simulink model "RPBSIDblocks"  (Simulink 7.8)
settings: Solver=ode45  StartTime=0.0  StopTime=10.0  RelTol=1e-3
values from neighbouring files (symbols this model uses):
  Du = 164.831638116    [GUST2data.mat]
  Dy = [1.80356893973  0; 0  1.68127100115]    [GUST2data.mat]
undefined symbols (not defined in the file or in its folder): W
libraries: cstblocks x1
(part 2 of 2)

== matlab function RPBSID (VARX) FAST-ARRAY ==
  data: ON input double; RESET input double; Ws output double; Fs1 output double; Fs2 output double; U input double; Y input double size=2; Wn output double; Zn output double; W parameter double; Du parameter double; Dy parameter double; ERR output double
function [Ws,Fs1,Fs2,Wn,Zn,ERR] = rpbsid(ON,RESET,U,Y,W,Du,Dy)
%RPBSID Closed-loop recursive predictor-based subspace identification (VARX)

% Input definitions
% U input sample
% Y output sample
% W weight matrix (from workspace)
% Du input scaling matrix from sigscale (from workspace)
% Dy output scaling matric from sigscale (from workspace)

% Common paremeters
r = 1;         % number if inpuh
l = 2;         % number of outpuh
m = l+r;
n = 7;         % number of states
Ts = 0.05;      % sample time

% Parameters for identification
p = 50;        % past window
f = 50;        % future window
noD = 0;       % no direct feedtrough
weight = 0;    % apply transformation filter

% Parameters for adaptive filters
lambda1 = 0.999; % initial forgetting factor (~= 1 - 2/window)
lambda2 = 0.999; % initial forgetting factor (~= 1 - 2/window)
lambda3 = 0.999; % initial forgetting factor (~= 1 - 2/window)
ireg1 = 100;     % initial regularisation
ireg2 = 1e-6;    % initial regularisation
ireg3 = 1e-6;    % initial regularisation
reg1 = 1;        % initial regularisation
tol = 1e-4;      % tolerance setting for resque (fast array)

% Initialization
startA = 3;

% Initialize if needed
persistent Plk Glk Ylk VARX VARX1 LK Pcd Pabk ABK CD U1 Y1 X X1 Z eta w k start saw
if isempty(Plk) || RESET
    % Initialisation of Markov estimation problem
    if noD
        Plk = zeros((p+1)*m+1,2*m+1);
        Glk = zeros(p*m,m);
        Ylk = ones(1,m);
        VARX = zeros(l,p*m);
        VARX1 = zeros(l,p*m);
        Z = zeros((p+1)*m,1);
        eta = zeros((p+1)*m,m);
    else
        Plk = zeros((p+2)*m+1,2*m+1);
        Glk = zeros((p+1)*m,m);
        Ylk = ones(1,m);
        VARX = zeros(l,(p+1)*m);
        VARX1 = zeros(l,p*m);
        Z = zeros((p+2)*m,1);
        eta = zeros((p+2)*m,m);
    end
    saw = 0;
    
    % Initialisation of the LambdaKappa
    LK = zeros(f*l,m*p);
    
    % Initialisation the estimate of ABK
    Pabk = (1/sqrt(ireg2)).*eye(n+r+l);
    ABK = [zeros(n) zeros(n,r) zeros(n,l)];
    
    if noD
        % Initialisation the estimate of CD
        Pcd = (1/sqrt(ireg3)).*eye(n);
        CD = zeros(l,n);
    else
        % Initialisation the estimate of CD and e
        Pcd = (1/sqrt(ireg3)).*eye(n+r);
        CD = [zeros(l,n) zeros(l,r)];
    end

    % Store vectors for next iteration
    Y1 = zeros(l,1);
    U1 = zeros(r,1);
    X1 = zeros(n,1);
    X = zeros(n,1);
    
    % Frequency grid
    w = logspace(-1,1,300);
    k = 1;
    start = 1;
end

% Start RPBSID iff ON is set
if ON > 0.5
    
    % Scale input and output
    U = diag(1./diag(Du))*U;
    Y = diag(1./diag(Dy))*Y;
    
    if (start < 0.5) || (k >= p)
        % Solve Markov estimation problem recursively
        if noD
            [VARX,Z,Plk,eta,Glk,Ylk,saw,ERR] = fastQR(Z,[U1; Y1],Y,VARX,Plk,lambda1,tol,eta,ireg1,reg1,Glk,Ylk,saw);
            VARX1 = VARX;
        else
            [VARX,Z,Plk,eta,Glk,Ylk,saw,ERR] = fastQR(Z,[Y1; U],Y,VARX,Plk,lambda1,tol,eta,ireg1,reg1,Glk,Ylk,saw);
            VARX1 = VARX(:,l+1:p*m+l);
        end
    else
        ERR = 0;
    end
    
    if (start < 0.5) || (k >= startA*p)
        % Construction of LambdaKappa
        LK = zeros(f*l,p*m);
        if ~weight
            for i = 0:f-1
                for h = 0:p-i-1
                    LK(i*l+(1:l),(i+h)*m+(1:m)) = VARX1(:,h*m+(1:m));
                end
            end
        else
            for i = 0:f-1
                for h = 0:p-i-1
                    LK(i*l+(1:l),(i+h)*m+(1:m)) = VARX1(:,h*m+(1:m));
                end
                if i ~= 0
                    for j = 0:i-1
                        LK(i*l+(1:l),:) = LK(i*l+(1:l),:) + VARX1(:,(p-i+j)*m+r+(1:l))*LK(j*l+(1:l),:);
                    end
                end
            end
        end
        
        % The estimation of the state vector
        if noD
            X = W*LK*Z(m+1:(p+1)*m,1);
        else
            X = W*LK*Z(m+l+1:(p+1)*m+l,1);
        end
    end
    
    if (start < 0.5) || (k >= startA*p+1)
        % The estimation of the system matrices
        if noD
            [CD,Pcd] = inverseQR(X1,Y1,CD,Pcd,lambda2);
            R1 = Y1-CD*X1;
        else
            [CD,Pcd] = inverseQR([X1; U1],Y1,CD,Pcd,lambda2);
            R1 = Y1-CD*[X1; U1];
        end
        [ABK,Pabk] = inverseQR([X1; U1; R1],X,ABK,Pabk,lambda3);
    end
        
    % Store vectors and matrices for next iteration
    if (start < 0.5) || (k >= startA*p)
        X1 = X;
    end
    Y1 = Y;
    U1 = U;
else
    ERR = 0;
end

% Store state-space matrices
A = ABK(:,1:n);
B = ABK(:,n+1:n+r)*diag(1./diag(Du));
C = Dy*CD(:,1:n);
if noD
    D = zeros(l,r);
else
    D = Dy*CD(:,n+1:end)*diag(1./diag(Du));
end
K = ABK(:,n+r+1:n+r+l);

% Calculate damping and frequencies
[Wn,Zn] = damp(A,Ts);

% Calculate frequency response
Ws = w(k);
Fs = real(abs(C*((exp(sqrt(complex(-1))*Ts*Ws*2*pi).*eye(n) - A)\B)+D));
Ws = log10(Ws);
if Fs(1) < 1e-5
    Fs1 = -100;
else
    Fs1 = 20*log10(Fs(1));
end
if Fs(2) < 1e-5
    Fs2 = -100;
else
    Fs2 = 20*log10(Fs(2));
end

% Update counter
if k >= length(w)
    start = 0;
    k = 1;
else
    k = k+1;
end

end % END RPBSID


function [theta,z,M,eta,G,Y,saw,ERR] = fastQR(z,u,y,theta,M,lambda,tol,eta,ireg,reg,G,Y,saw)
%FASTQR Fast Recursive Least Squares (fast array QR)

n = length(u);
p = (length(z)/n - 1);
if M(1,1) == 0
    M(1,1) = 1;
    M(2:n+1,2:n+1) = diag((sqrt(lambda^p)/sqrt(ireg)).*ones(n,1));
    M(p*n+2:(p+1)*n+1,n+2:2*n+1) = diag((1/sqrt(ireg)).*ones(n,1));
end

% Do reg update
if saw > p-0.5;
    saw = 1;
    eta = [eta(n+1:end,:); sqrt((1-lambda^p)*reg).*eye(n)];
else
    saw = saw + 1;
    eta = [eta(n+1:end,:); zeros(n)];
end

G1 = M(2+n:end,1);
Y1 = M(1,1);
for j = 1:n
    M(1,1) = Y(1,j);
    M(2:end,2:end) = M(2:end,2:end);
    M(1,2:end) = eta(:,j)'*M(2:end,2:end);
    M(2:1+p*n,1) = G(1:end,j);
    M(2+p*n:end,1) = zeros(n,1);
    for i = 2:size(M,2)
        if i > (size(M,2)-n)
            % determine Givens rotation parameters
            if M(1,i) ~= 0
                % determine Givens rotation parameters
                rho = M(1,i)/M(1,1);
                c = sqrt(1+abs(rho)^2);
                
                % apply givens rotation using mixed-downdating
                M(:,1) = (M(:,1) + rho.*M(:,i))./c;
                M(:,i) = (-rho).*M(:,1) + c.*M(:,i);
            end
        else
            % determine hyperbolic rotation parameters
            if abs(M(i,i)) > abs(M(i,1))
                if M(i,1) ~= 0
                    % apply hyperbolic rotation using orthogonal-diagonal method
                    % method (numerically stable)
                    x1 = M(:,1) - M(:,i);
                    y1 = M(:,1) + M(:,i);
                    x2 = 0.5.*sqrt(-y1(i)/x1(i)).*x1;
                    y2 = 0.5.*sqrt(-x1(i)/y1(i)).*y1;
                    M(:,1) = x2 + y2;
                    M(:,i) = y2 - x2;
                end
            else
                M = zeros((p+1)*n+1,2*n+1);
                M(1,1) = 1;
                M(2:n+1,2:n+1) = diag((sqrt(lambda^p)/sqrt(ireg)).*ones(n,1));
                M(p*n+2:(p+1)*n+1,n+2:2*n+1) = diag((1/sqrt(ireg)).*ones(n,1));
                G = zeros(p*n,n);
                Y = ones(1,n);
                ERR = norm(M(1,2:n+1));
                z = zeros((p+1)*n,1);
                return
            end
        end
    end
    Y(1,j) = M(1,1);
    G(1:end,j) = M(n+2:end,1);
end

% Do data update
z = [z(n+1:end); u];
M(1,1) = Y1;
M(2:end,2:end) = M(2:end,2:end)./sqrt(lambda);
M(1,2:end) = z'*M(2:end,2:end);
M(2:1+p*n,1) = G1;
M(2+p*n:end,1) = zeros(n,1);
for i = 2:size(M,2)
    if i > (size(M,2)-n)
        % determine Givens rotation parameters
        if M(1,i) ~= 0
            % determine Givens rotation parameters
            rho = M(1,i)/M(1,1);
            c = sqrt(1+abs(rho)^2);
            
            % apply givens rotation using mixed-downdating
            M(:,1) = (M(:,1) + rho.*M(:,i))./c;
            M(:,i) = (-rho).*M(:,1) + c.*M(:,i);
        end
    else
        % determine hyperbolic rotation parameters
        if abs(M(i,i)) > abs(M(i,1))
            if M(i,1) ~= 0
                % apply hyperbolic rotation using orthogonal-diagonal method
                % method (numerically stable)
                x1 = M(:,1) - M(:,i);
                y1 = M(:,1) + M(:,i);
                x2 = 0.5.*sqrt(-y1(i)/x1(i)).*x1;
                y2 = 0.5.*sqrt(-x1(i)/y1(i)).*y1;
                M(:,1) = x2 + y2;
                M(:,i) = y2 - x2;
            end
        else
            M = zeros((p+1)*n+1,2*n+1);
            M(1,1) = 1;
            M(2:n+1,2:n+1) = diag((sqrt(lambda^p)/sqrt(ireg)).*ones(n,1));
            M(p*n+2:(p+1)*n+1,n+2:2*n+1) = diag((1/sqrt(ireg)).*ones(n,1));
            G = zeros(p*n,n);
            Y = ones(1,n);
            ERR = norm(M(1,2:n+1));
            z = zeros((p+1)*n,1);
            return
        end
    end
end

ERR = norm(M(1,2:n+1));
if ERR < tol
    E = y - theta*z(n+1:end);
    theta = theta + E*(M(n+2:end,1)/M(1,1))';
else
    M = zeros((p+1)*n+1,2*n+1);
    M(1,1) = 1;
    M(2:n+1,2:n+1) = diag((sqrt(lambda^p)/sqrt(ireg)).*ones(n,1));
    M(p*n+2:(p+1)*n+1,n+2:2*n+1) = diag((1/sqrt(ireg)).*ones(n,1));
    G = zeros(p*n,n);
    Y = ones(1,n);
    z = zeros((p+1)*n,1);
end
end

function [theta,P,R] = inverseQR(z,y,theta,P,lambda)
%INVERSEQR Square-Root Recursive Least Squares update (inverse QR)

[mz,nz] = size(z);
zp = z'*P;
M = [eye(nz) (zp)./sqrt(lambda); zeros(mz,nz) P./sqrt(lambda)];
for i = (size(P,2)+nz):-1:2
    % determine Givens rotation parameters
    if M(1,i) == 0
    elseif M(1,1) == 0
        % swap
        h = M(:,i);
        M(:,i) = -M(:,1);
        M(:,1) = h;
    else
        % determine Givens rotation parameters
        rho = M(1,i)/M(1,1);
        c = sqrt(1+abs(rho)^2);
        
        % apply givens rotation using mixed-downdating (more numeric stable)
        M(:,1) = (M(:,1) + rho.*M(:,i))./c;
        M(:,i) = -rho.*M(:,1) + c.*M(:,i);
    end
end
G = M(nz+1:end,1:nz)/M(1:nz,1:nz);
P = M(nz+1:end,nz+1:end);
E = y - theta*z;
theta = theta + E*G';
if nargout == 3
    R = norm(y - theta*z);
end
end


function [wn,z] = damp(a,Ts)
%DAMP  Natural frequency and damping

% Calculate eigenvalues
r = eig(a);
[~,I] = sort(real(r));
r = r(I);

% Discrete: compute equivalent S-plane poles
if any(r) == 0
    z = zeros(size(r));
    wn = zeros(size(r));
else
    s = log(r)/Ts;
    f = abs(s);
    wn = f;
    z = -real(s)./f;
end
end

%% UNCOMMENT THE LATTER FOR OLDER MATLAB VERSIONS

% function y = log10(x)
% %LOG10  Common (base 10) logarithm.
% y = log(x)/log(10);
% end

% function E = eig(A)
% % Compute eigenvalues of matrix
% tol = 1e-4;
% maxit = 20;
% n = size(A,1);
% C = complex(A,zeros(n));
% A1 = C(n,n);
% E = complex(zeros(n,1),zeros(n,1));
% I = eye(n);
% for k2 = n:-1:2
%     k = 1;
%     brk = 0;
%     while k <= maxit && brk <= 0.5
%         mu = qrshift(C(k2+(-1:0),k2+(-1:0)));
%         M = (C - mu(1).*I);
%         [Q,R] = qr(M);
%         C = (R*Q + mu(1).*I);
%         if abs(abs(A1)-abs(C(k2,k2))) < tol
%             brk = 1;
%             A1 = C(k2-1,k2-1);
%         else
%             A1 = C(k2,k2);
%         end
%         k = k+1;
%     end
%     E(k2) = C(k2,k2);
%     C(k2,1:n) = 0;
%     C(1:n,k2) = 0;
%     I(k2,k2) = 0;
% end
% E(1) = C(1,1);
% E = sort(E);
% end

% function mu = qrshift(A)
% % Compute the Wilkinson double shift
% 
% trA = A(1,1) + A(2,2);
% detA =  A(1,1)*A(2,2) - A(1,2)*A(2,1);
% 
% mu1 = 0.5*(trA + sqrt(trA^2-4*detA));
% mu2 = 0.5*(trA - sqrt(trA^2-4*detA));
% if abs(abs(A(2,2)) - abs(mu1)) < abs(abs(A(2,2)) - abs(mu2))
%     mu = mu1;
% else
%     mu = mu2;
% end
% end

== matlab function RPBSID (VARMAX) FAST-ARRAY ==
  data: ON input double; RESET input double; Ws output double; Fs1 output double; Fs2 output double; U input double; Y input double size=2; Wn output double; Zn output double; W parameter double; Du parameter double; Dy parameter double; ERR output double
function [Ws,Fs1,Fs2,Wn,Zn,ERR] = rpbsid(ON,RESET,U,Y,W,Du,Dy)
%RPBSID Closed-loop recursive predictor-based subspace identification (VARX)

% Input definitions
% U input sample
% Y output sample
% W weight matrix (from workspace)
% Du input scaling matrix from sigscale (from workspace)
% Dy output scaling matric from sigscale (from workspace)

% Common paremeters
r = 1;         % number if inpuh
l = 2;         % number of outpuh
m = 2*l+r;
n = 7;         % number of states
Ts = 0.05;      % sample time

% Parameters for identification
p = 50;        % past window
f = 50;        % future window
noD = 0;       % no direct feedtrough
weight = 0;    % apply transformation filter

% Parameters for adaptive filters
lambda1 = 0.999; % initial forgetting factor (~= 1 - 2/window)
lambda2 = 0.999; % initial forgetting factor (~= 1 - 2/window)
lambda3 = 0.999; % initial forgetting factor (~= 1 - 2/window)
ireg1 = 100;     % initial regularisation
ireg2 = 1e-6;    % initial regularisation
ireg3 = 1e-6;    % initial regularisation
reg1 = 1;        % initial regularisation
tol = 1e-4;      % tolerance setting for resque (fast array)

% Initialization
startA = 3;

% Initialize if needed
persistent Plk Glk Ylk VARX VARX1 LK Pcd Pabk ABK CD U1 Y1 E1 X X1 Z eta w k start saw
if isempty(Plk) || RESET
    % Initialisation of Markov estimation problem
    if noD
        Plk = zeros((p+1)*m+1,2*m+1);
        Glk = zeros(p*m,m);
        Ylk = ones(1,m);
        VARX = zeros(l,p*m);
        VARX1 = zeros(l,p*m);
        Z = zeros((p+1)*m,1);
        eta = zeros((p+1)*m,m);
    else
        Plk = zeros((p+2)*m+1,2*m+1);
        Glk = zeros((p+1)*m,m);
        Ylk = ones(1,m);
        VARX = zeros(l,(p+1)*m);
        VARX1 = zeros(l,p*m+r);
        Z = zeros((p+2)*m,1);
        eta = zeros((p+2)*m,m);
    end
    saw = 0;
    
    % Initialisation of the LambdaKappa
    LK = zeros(f*l,m*p);
    
    % Initialisation the estimate of ABK
    Pabk = (1/sqrt(ireg2)).*eye(n+r+l);
    ABK = [zeros(n) zeros(n,r) zeros(n,l)];
    
    if noD
        % Initialisation the estimate of CD
        Pcd = (1/sqrt(ireg3)).*eye(n);
        CD = zeros(l,n);
    else
        % Initialisation the estimate of CD and e
        Pcd = (1/sqrt(ireg3)).*eye(n+r);
        CD = [zeros(l,n) zeros(l,r)];
    end

    % Store vectors for next iteration
    Y1 = zeros(l,1);
    U1 = zeros(r,1);
    X1 = zeros(n,1);
    X = zeros(n,1);
    E1 = zeros(l,1);
    
    % Frequency grid
    w = logspace(-1,1,300);
    k = 1;
    start = 1;
end

% Start RPBSID iff ON is set
if ON > 0.5
    
    % Scale input and output
    U = diag(1./diag(Du))*U;
    Y = diag(1./diag(Dy))*Y;
    
    if (start < 0.5) || (k >= p)
        % Solve Markov estimation problem recursively
        if noD
            [VARX,Z,Plk,eta,Glk,Ylk,saw,ERR] = fastQR(Z,[U1; Y1; E1],Y,VARX,Plk,lambda1,tol,eta,ireg1,reg1,Glk,Ylk,saw);
            VARX1 = VARX;
            E1 = Y - VARX1*Z(m+1:(p+1)*m,1);
        else
            [VARX,Z,Plk,eta,Glk,Ylk,saw,ERR] = fastQR(Z,[Y1; E1; U],Y,VARX,Plk,lambda1,tol,eta,ireg1,reg1,Glk,Ylk,saw);
            VARX1 = VARX(:,2*l+1:(p+1)*m);
            E1 = Y - VARX1*Z(m+2*l+1:(p+2)*m,1);
        end
    else
        ERR = 0;
    end
    
    if (start < 0.5) || (k >= startA*p)
        % Construction of LambdaKappa
        LK = zeros(f*l,p*m);
        if ~weight
            for i = 0:f-1
                for h = 0:p-i-1
                    LK(i*l+(1:l),(i+h)*m+(1:m)) = VARX1(:,h*m+(1:m));
                end
            end
        else
            for i = 0:f-1
                for h = 0:p-i-1
                    LK(i*l+(1:l),(i+h)*m+(1:m)) = VARX1(:,h*m+(1:m));
                end
                if i ~= 0
                    for j = 0:i-1
                        LK(i*l+(1:l),:) = LK(i*l+(1:l),:) + VARX1(:,(p-i+j)*m+r+(1:l))*LK(j*l+(1:l),:);
                    end
                end
            end
        end
        
        % The estimation of the state vector
        if noD
            X = W*LK*Z(m+1:(p+1)*m,1);
        else
            X = W*LK*Z(m+l+1:(p+1)*m+l,1);
        end
    end
    
    if (start < 0.5) || (k >= startA*p+1)
        % The estimation of the system matrices
        if noD
            [CD,Pcd] = inverseQR(X1,Y1,CD,Pcd,lambda2);
            R1 = Y1-CD*X1;
        else
            [CD,Pcd] = inverseQR([X1; U1],Y1,CD,Pcd,lambda2);
            R1 = Y1-CD*[X1; U1];
        end
        [ABK,Pabk] = inverseQR([X1; U1; R1],X,ABK,Pabk,lambda3);
    end
        
    % Store vectors and matrices for next iteration
    if (start < 0.5) || (k >= startA*p)
        X1 = X;
    end
    Y1 = Y;
    U1 = U;
else
    ERR = 0;
end

% Store state-space matrices
A = ABK(:,1:n);
B = ABK(:,n+1:n+r)*diag(1./diag(Du));
C = Dy*CD(:,1:n);
if noD
    D = zeros(l,r);
else
    D = Dy*CD(:,n+1:end)*diag(1./diag(Du));
end
K = ABK(:,n+r+1:n+r+l);

% Calculate damping and frequencies
[Wn,Zn] = damp(A,Ts);

% Calculate frequency response
Ws = w(k);
Fs = real(abs(C*((exp(sqrt(complex(-1))*Ts*Ws*2*pi).*eye(n) - A)\B)+D));
Ws = log10(Ws);
if Fs(1) < 1e-5
    Fs1 = -100;
else
    Fs1 = 20*log10(Fs(1));
end
if Fs(2) < 1e-5
    Fs2 = -100;
else
    Fs2 = 20*log10(Fs(2));
end

% Update counter
if k >= length(w)
    start = 0;
    k = 1;
else
    k = k+1;
end

end % END RPBSID


function [theta,z,M,eta,G,Y,saw,ERR] = fastQR(z,u,y,theta,M,lambda,tol,eta,ireg,reg,G,Y,saw)
%FASTQR Fast Recursive Least Squares (fast array QR)

n = length(u);
p = (length(z)/n - 1);
if M(1,1) == 0
    M(1,1) = 1;
    M(2:n+1,2:n+1) = diag((sqrt(lambda^p)/sqrt(ireg)).*ones(n,1));
    M(p*n+2:(p+1)*n+1,n+2:2*n+1) = diag((1/sqrt(ireg)).*ones(n,1));
end

% Do reg update
if saw > p-0.5;
    saw = 1;
    eta = [eta(n+1:end,:); sqrt((1-lambda^p)*reg).*eye(n)];
else
    saw = saw + 1;
    eta = [eta(n+1:end,:); zeros(n)];
end

G1 = M(2+n:end,1);
Y1 = M(1,1);
for j = 1:n
    M(1,1) = Y(1,j);
    M(2:end,2:end) = M(2:end,2:end);
    M(1,2:end) = eta(:,j)'*M(2:end,2:end);
    M(2:1+p*n,1) = G(1:end,j);
    M(2+p*n:end,1) = zeros(n,1);
    for i = 2:size(M,2)
        if i > (size(M,2)-n)
            % determine Givens rotation parameters
            if M(1,i) ~= 0
                % determine Givens rotation parameters
                rho = M(1,i)/M(1,1);
                c = sqrt(1+abs(rho)^2);
                
                % apply givens rotation using mixed-downdating
                M(:,1) = (M(:,1) + rho.*M(:,i))./c;
                M(:,i) = (-rho).*M(:,1) + c.*M(:,i);
            end
        else
            % determine hyperbolic rotation parameters
            if abs(M(i,i)) > abs(M(i,1))
                if M(i,1) ~= 0
                    % apply hyperbolic rotation using orthogonal-diagonal method
                    % method (numerically stable)
                    x1 = M(:,1) - M(:,i);
                    y1 = M(:,1) + M(:,i);
                    x2 = 0.5.*sqrt(-y1(i)/x1(i)).*x1;
                    y2 = 0.5.*sqrt(-x1(i)/y1(i)).*y1;
                    M(:,1) = x2 + y2;
                    M(:,i) = y2 - x2;
                end
            else
                M = zeros((p+1)*n+1,2*n+1);
                M(1,1) = 1;
                M(2:n+1,2:n+1) = diag((sqrt(lambda^p)/sqrt(ireg)).*ones(n,1));
                M(p*n+2:(p+1)*n+1,n+2:2*n+1) = diag((1/sqrt(ireg)).*ones(n,1));
                G = zeros(p*n,n);
                Y = ones(1,n);
                ERR = norm(M(1,2:n+1));
                z = zeros((p+1)*n,1);
                return
            end
        end
    end
    Y(1,j) = M(1,1);
    G(1:end,j) = M(n+2:end,1);
end

% Do data update
z = [z(n+1:end); u];
M(1,1) = Y1;
M(2:end,2:end) = M(2:end,2:end)./sqrt(lambda);
M(1,2:end) = z'*M(2:end,2:end);
M(2:1+p*n,1) = G1;
M(2+p*n:end,1) = zeros(n,1);
for i = 2:size(M,2)
    if i > (size(M,2)-n)
        % determine Givens rotation parameters
        if M(1,i) ~= 0
            % determine Givens rotation parameters
            rho = M(1,i)/M(1,1);
            c = sqrt(1+abs(rho)^2);
            
            % apply givens rotation using mixed-downdating
            M(:,1) = (M(:,1) + rho.*M(:,i))./c;
            M(:,i) = (-rho).*M(:,1) + c.*M(:,i);
        end
    else
        % determine hyperbolic rotation parameters
        if abs(M(i,i)) > abs(M(i,1))
            if M(i,1) ~= 0
                % apply hyperbolic rotation using orthogonal-diagonal method
                % method (numerically stable)
                x1 = M(:,1) - M(:,i);
                y1 = M(:,1) + M(:,i);
                x2 = 0.5.*sqrt(-y1(i)/x1(i)).*x1;
                y2 = 0.5.*sqrt(-x1(i)/y1(i)).*y1;
                M(:,1) = x2 + y2;
                M(:,i) = y2 - x2;
            end
        else
            M = zeros((p+1)*n+1,2*n+1);
            M(1,1) = 1;
            M(2:n+1,2:n+1) = diag((sqrt(lambda^p)/sqrt(ireg)).*ones(n,1));
            M(p*n+2:(p+1)*n+1,n+2:2*n+1) = diag((1/sqrt(ireg)).*ones(n,1));
            G = zeros(p*n,n);
            Y = ones(1,n);
            ERR = norm(M(1,2:n+1));
            z = zeros((p+1)*n,1);
            return
        end
    end
end

ERR = norm(M(1,2:n+1));
if ERR < tol
    E = y - theta*z(n+1:end);
    theta = theta + E*(M(n+2:end,1)/M(1,1))';
else
    M = zeros((p+1)*n+1,2*n+1);
    M(1,1) = 1;
    M(2:n+1,2:n+1) = diag((sqrt(lambda^p)/sqrt(ireg)).*ones(n,1));
    M(p*n+2:(p+1)*n+1,n+2:2*n+1) = diag((1/sqrt(ireg)).*ones(n,1));
    G = zeros(p*n,n);
    Y = ones(1,n);
    z = zeros((p+1)*n,1);
end
end

function [theta,P,R] = inverseQR(z,y,theta,P,lambda)
%INVERSEQR Square-Root Recursive Least Squares update (inverse QR)

[mz,nz] = size(z);
zp = z'*P;
M = [eye(nz) (zp)./sqrt(lambda); zeros(mz,nz) P./sqrt(lambda)];
for i = (size(P,2)+nz):-1:2
    % determine Givens rotation parameters
    if M(1,i) == 0
    elseif M(1,1) == 0
        % swap
        h = M(:,i);
        M(:,i) = -M(:,1);
        M(:,1) = h;
    else
        % determine Givens rotation parameters
        rho = M(1,i)/M(1,1);
        c = sqrt(1+abs(rho)^2);
        
        % apply givens rotation using mixed-downdating (more numeric stable)
        M(:,1) = (M(:,1) + rho.*M(:,i))./c;
        M(:,i) = -rho.*M(:,1) + c.*M(:,i);
    end
end
G = M(nz+1:end,1:nz)/M(1:nz,1:nz);
P = M(nz+1:end,nz+1:end);
E = y - theta*z;
theta = theta + E*G';
if nargout == 3
    R = norm(y - theta*z);
end
end


function [wn,z] = damp(a,h)
%DAMP  Natural frequency and damping

% Calculate eigenvalues
r = eig(a);
[~,I] = sort(real(r));
r = r(I);

% Discrete: compute equivalent S-plane poles
if any(r) == 0
    z = zeros(size(r));
    wn = zeros(size(r));
else
    s = log(r)/h;
    f = abs(s);
    wn = f;
    z = -real(s)./f;
end
end

%% UNCOMMENT THE LATTER FOR OLDER MATLAB VERSIONS

% function y = log10(x)
% %LOG10  Common (base 10) logarithm.
% y = log(x)/log(10);
% end

% function E = eig(A)
% % Compute eigenvalues of matrix
% tol = 1e-4;
% maxit = 20;
% n = size(A,1);
% C = complex(A,zeros(n));
% A1 = C(n,n);
% E = complex(zeros(n,1),zeros(n,1));
% I = eye(n);
% for k2 = n:-1:2
%     k = 1;
%     brk = 0;
%     while k <= maxit && brk <= 0.5
%         mu = qrshift(C(k2+(-1:0),k2+(-1:0)));
%         M = (C - mu(1).*I);
%         [Q,R] = qr(M);
%         C = (R*Q + mu(1).*I);
%         if abs(abs(A1)-abs(C(k2,k2))) < tol
%             brk = 1;
%             A1 = C(k2-1,k2-1);
%         else
%             A1 = C(k2,k2);
%         end
%         k = k+1;
%     end
%     E(k2) = C(k2,k2);
%     C(k2,1:n) = 0;
%     C(1:n,k2) = 0;
%     I(k2,k2) = 0;
% end
% E(1) = C(1,1);
% E = sort(E);
% end

% function mu = qrshift(A)
% % Compute the Wilkinson double shift
% 
% trA = A(1,1) + A(2,2);
% detA =  A(1,1)*A(2,2) - A(1,2)*A(2,1);
% 
% mu1 = 0.5*(trA + sqrt(trA^2-4*detA));
% mu2 = 0.5*(trA - sqrt(trA^2-4*detA));
% if abs(abs(A(2,2)) - abs(mu1)) < abs(abs(A(2,2)) - abs(mu2))
%     mu = mu1;
% else
%     mu = mu2;
% end
% end

== matlab function Pulse Counter ==
  data: Y input double; freq output double
function freq = pulse(Y)
%PULSE COUNTER

% Sample time
Ts = 0.001;
init = 100/Ts;

% Initialize if needed
persistent T P k
if isempty(T)
    k = 1;
    P = 0;
    T = init;
end

if Y < 5
    if P > 0.5
        T = k;
        P = 0;
        k = 1;
    end
else
    if P < 0.5
        P = 1;
    end    
end
if k*Ts < 100
    k = k + 1;
end
freq = 1/(T*Ts); % frequency in Hertz
% freq = 0.159155*freq; % convert to rad/sec
